simulink model "ebike"  (R2016a)
settings: Solver=ode3  StartTime=0.0  StopTime=1  FixedStep=0.001  MaxStep=0.001  MinStep=0.001  RelTol=1e-3
undefined symbols (not defined in the file or in its folder): RPM_motor_power
libraries: simulink x1
settings Model: Creator=stwei  LastModifiedBy=Aparajith Sridharan
settings DataIOCC: LimitDataPoints=on  SaveFormat=Array  SaveOutput=off  ReturnWorkspaceOutputs=on
settings OptimizationCC: ExpressionDepthLimit=2147483647
settings DebuggingCC: UnderspecifiedInitializationDetection=Classic  MergeDetectMultiDrivingBlocksExec=none  SolverPrmCheckMsg=warning  FcnCallInpInsideContextMsg=UseLocalSettings  StateNameClashWarn=warning
settings HardwareCC: ProdBitPerPointer=32  ProdLargestAtomicFloat=None  ProdIntDivRoundTo=Undefined  ProdEndianess=Unspecified  ProdWordSize=32  ProdHWDeviceType=32-bit Generic
settings ModelReferenceCC: PropagateSignalLabelsOutOfModel=off
settings GRTTargetCC: CombineOutputUpdateFcns=off  GRTInterface=on
settings ConfigComp: CovModelRefEnable=Off

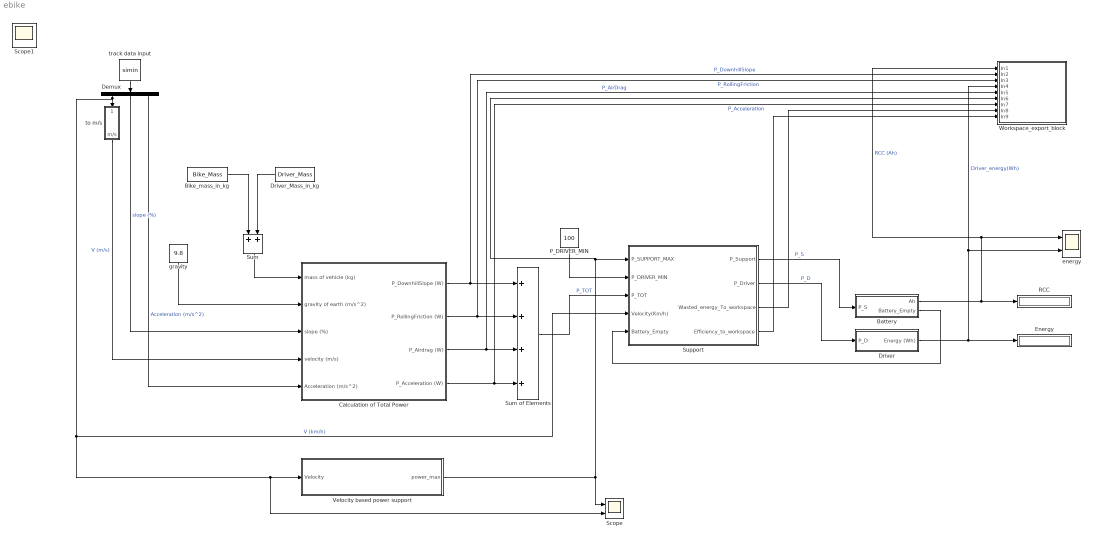
== system ebike ==
  Battery : Subsystem
  Bike_mass_in_kg : FromWorkspace  VariableName=Bike_Mass  SampleTime=0
  Calculation of Total Power : Subsystem
  Demux : Demux  Outputs=3
  Driver : Subsystem
  Driver_Mass_in_kg : FromWorkspace  VariableName=Driver_Mass  SampleTime=0
  Energy : Display
  P_DRIVER_MIN : Constant  Value=100
  RCC : Display
  Scope : Scope  NumInputPorts=2
  "Sum " : Sum
  Sum of Elements : Sum  Inputs=++++
  Support : Subsystem
  Velocity based power support : Subsystem
  Workspace_export_block : Subsystem
  energy : Scope  NumInputPorts=2
  gravity : Constant  Value=9.8
  to m/s : Subsystem
  track data input : FromWorkspace  VariableName=simin  SampleTime=0  OutputAfterFinalValue=Setting to zero
  Scope1 : Scope
  wires:
  P_DRIVER_MIN/1 -> Support/2(P_DRIVER_MIN)
  Support/2(P_Driver) -> Driver/1(P_D)  "P_D"
  Battery/1(Ah) -> RCC/1, energy/1, Workspace_export_block/1(In1)  "RCC (Ah)"
  track data input/1 -> Demux/1
  Demux/1 -> Support/4(Velocity(Km/h)), Scope/2, Velocity based power support/1(Velocity), to m/s/1(km/h)  "V (km/h)"
  Demux/2 -> Calculation of Total Power/3(slope (%))  "slope (%)"
  to m/s/1(m/s) -> Calculation of Total Power/4(velocity (m/s))  "V (m/s)"
  Sum of Elements/1 -> Support/3(P_TOT)  "P_TOT"
  Calculation of Total Power/1(P_DownhillSlope (W)) -> Workspace_export_block/2(In2), Sum of Elements/1  "P_DownhillSlope"
  Calculation of Total Power/2(P_RollingFriction (W)) -> Workspace_export_block/3(In3), Sum of Elements/2  "P_RollingFriction"
  Calculation of Total Power/3(P_Airdrag (W)) -> Workspace_export_block/5(In5), Sum of Elements/3  "P_AirDrag"
  Calculation of Total Power/4(P_Acceleration (W)) -> Workspace_export_block/7(In7), Sum of Elements/4  "P_Acceleration"
  gravity/1 -> Calculation of Total Power/2("gravity of earth (m/s^2) ")
  "Sum "/1 -> Calculation of Total Power/1(mass of vehicle (kg))
  Driver_Mass_in_kg/1 -> "Sum "/2
  Bike_mass_in_kg/1 -> "Sum "/1
  Demux/3 -> Calculation of Total Power/5(Acceleration (m/s^2))  "Acceleration (m/s^2)"
  Velocity based power support/1(power_max) -> Workspace_export_block/6(In6), Support/1(P_SUPPORT_MAX), Scope/1
  Driver/1(Energy (Wh)) -> Workspace_export_block/4(In4), energy/2, Energy/1  "Driver_energy(Wh)"
  Support/1(P_Support) -> Battery/1(P_S)  "P_S"
  Battery/2(Battery_Empty) -> Support/5(Battery_Empty)
  Support/3(Wasted_energy_To_workspace) -> Workspace_export_block/8(In8)
  Support/4(Efficiency_to_workspace) -> Workspace_export_block/9(In9)

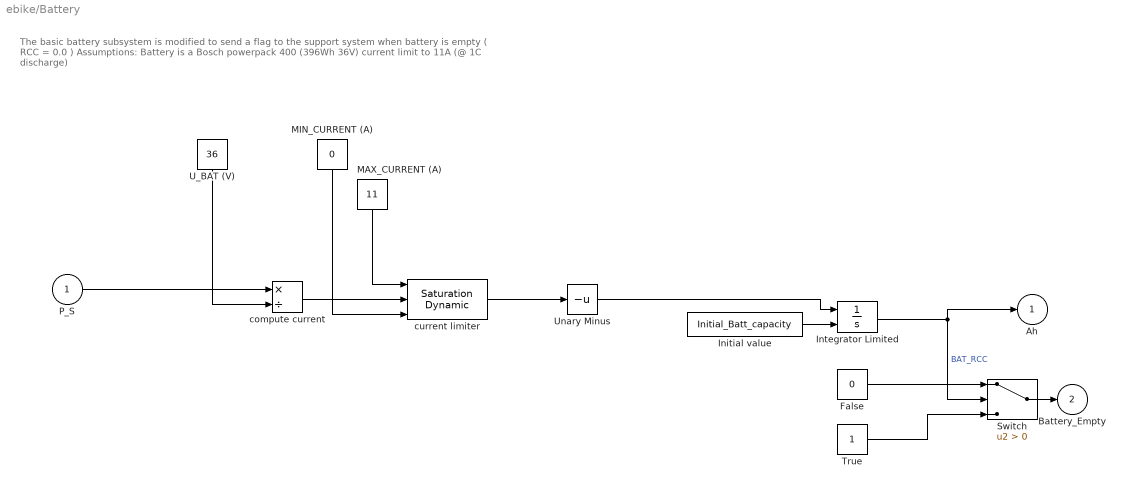
== system ebike/Battery ==
  note: The basic battery subsystem is modified to send a flag to the support system when battery is empty ( RCC = 0.0 )
      | Assumptions:
      | Battery is a Bosch powerpack 400 (396Wh 36V)
      | current limit to 11A (@ 1C discharge)
  P_S : Inport
  False : Constant  Value=0
  "Initial value " : FromWorkspace  VariableName=Initial_Batt_capacity  SampleTime=0
  Integrator Limited : Integrator  InitialConditionSource=external  LimitOutput=on  UpperSaturationLimit=11  LowerSaturationLimit=0
  MAX_CURRENT (A) : Constant  Value=11
  MIN_CURRENT (A) : Constant  Value=0
  Switch : Switch  Criteria=u2 > Threshold
  True : Constant
  U_BAT (V) : Constant  Value=36
  Unary Minus : UnaryMinus
  compute current : Product  Inputs=*/
  current limiter : simulink/Discontinuities/Saturation Dynamic  OutMin=[]  OutMax=[]  OutDataTypeStr=Inherit: Same as second input  OutDataType=fixdt(1, 16)  OutScaling=2^-10  DoSatur=on
  Ah : Outport
  Battery_Empty : Outport  Port=2
  wires:
  U_BAT (V)/1 -> compute current/2
  Integrator Limited/1 -> Ah/1, Switch/2  "BAT_RCC"
  current limiter/1 -> Unary Minus/1
  compute current/1 -> current limiter/2
  MAX_CURRENT (A)/1 -> current limiter/1
  MIN_CURRENT (A)/1 -> current limiter/3
  Unary Minus/1 -> Integrator Limited/1
  P_S/1 -> compute current/1
  "Initial value "/1 -> Integrator Limited/2
  Switch/1 -> Battery_Empty/1
  False/1 -> Switch/1
  True/1 -> Switch/3

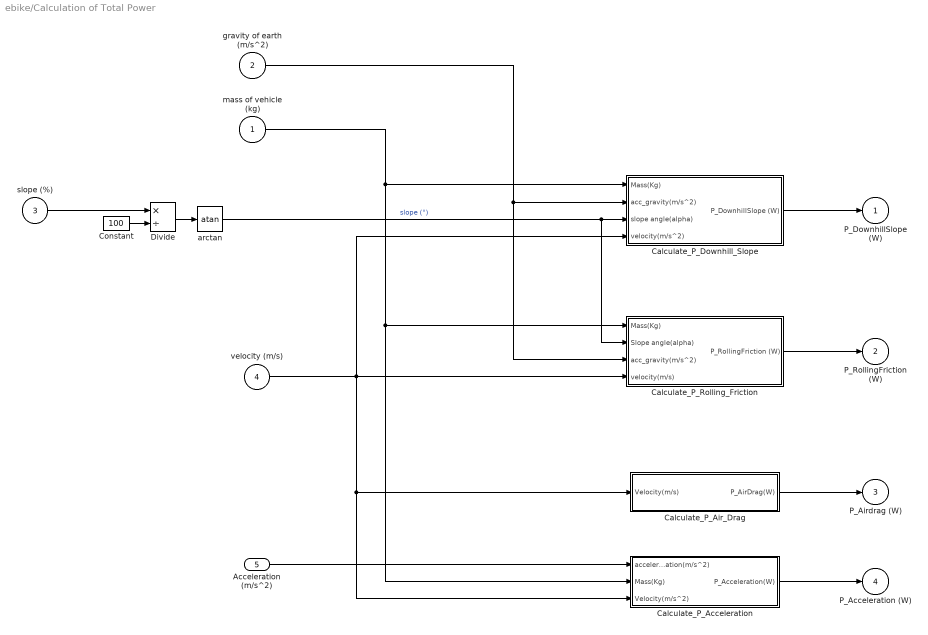
== system ebike/Calculation of Total Power ==
  mass of vehicle (kg) : Inport
  "gravity of earth (m/s^2) " : Inport  Port=2
  slope (%) : Inport  Port=3
  velocity (m/s) : Inport  Port=4
  Acceleration (m/s^2) : Inport  Port=5
  Calculate_P_Acceleration : Subsystem
  Calculate_P_Air_Drag : Subsystem
  Calculate_P_Downhill_Slope : Subsystem
  Calculate_P_Rolling_Friction : Subsystem
  Constant : Constant  Value=100
  Divide : Product  Inputs=*/
  arctan : Trigonometry  Operator=atan
  P_DownhillSlope (W) : Outport
  P_RollingFriction (W) : Outport  Port=2
  P_Airdrag (W) : Outport  Port=3
  P_Acceleration (W) : Outport  Port=4
  wires:
  mass of vehicle (kg)/1 -> Calculate_P_Downhill_Slope/1(Mass(Kg)), Calculate_P_Acceleration/2(Mass(Kg)), Calculate_P_Rolling_Friction/1(Mass(Kg))
  "gravity of earth (m/s^2) "/1 -> Calculate_P_Downhill_Slope/2(acc_gravity(m/s^2)), Calculate_P_Rolling_Friction/3(acc_gravity(m/s^2))
  velocity (m/s)/1 -> Calculate_P_Rolling_Friction/4(velocity(m/s)), Calculate_P_Air_Drag/1(Velocity(m/s)), Calculate_P_Acceleration/3(Velocity(m/s^2)), Calculate_P_Downhill_Slope/4(velocity(m/s^2))
  Calculate_P_Downhill_Slope/1(P_DownhillSlope (W)) -> P_DownhillSlope (W)/1
  arctan/1 -> Calculate_P_Rolling_Friction/2(Slope angle(alpha)), Calculate_P_Downhill_Slope/3(slope angle(alpha))  "slope (°)"
  Divide/1 -> arctan/1
  slope (%)/1 -> Divide/1
  Constant/1 -> Divide/2
  Acceleration (m/s^2)/1 -> Calculate_P_Acceleration/1(acceleration(m/s^2))
  Calculate_P_Acceleration/1("P_Acceleration(W) ") -> P_Acceleration (W)/1
  Calculate_P_Rolling_Friction/1(P_RollingFriction (W)) -> P_RollingFriction (W)/1
  Calculate_P_Air_Drag/1("P_AirDrag(W) ") -> P_Airdrag (W)/1

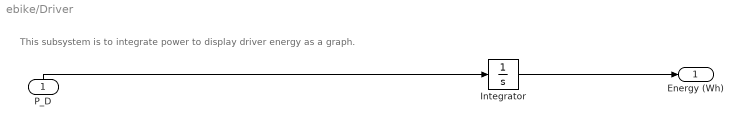
== system ebike/Driver ==
  note: This subsystem is to integrate power to display driver energy as a graph.
  P_D : Inport
  "Integrator " : Integrator  UpperSaturationLimit=400  LowerSaturationLimit=0
  Energy (Wh) : Outport
  wires:
  "Integrator "/1 -> Energy (Wh)/1
  P_D/1 -> "Integrator "/1

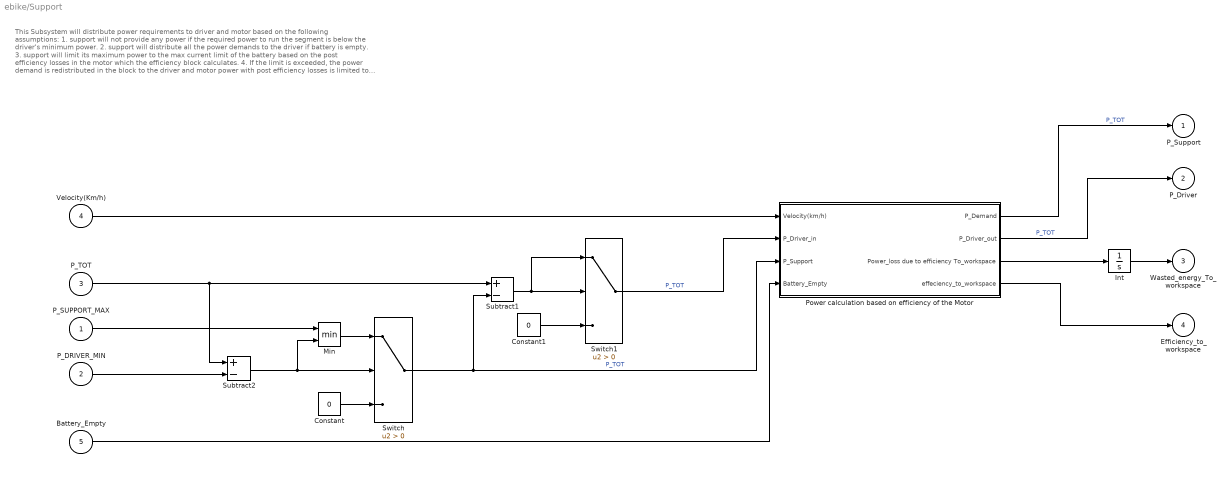
== system ebike/Support ==
  note: This Subsystem will distribute power requirements to driver and motor based on the following assumptions:
      | 1. support will not provide any power if the required power to run the segment is below the driver's minimum power.
      | 2. support will distribute all the power demands to the driver if battery is empty.
      | 3. support will limit its maximum power to the max current limit of the battery based on the post efficiency losses in the motor which the efficiency block calculates.
      | 4. If the limit is exceeded, the power demand is redistributed in the block to the driver and motor power with post efficiency losses is limited to max current limit of battery subsystem.
  P_SUPPORT_MAX : Inport
  P_DRIVER_MIN : Inport  Port=2
  P_TOT : Inport  Port=3
  Velocity(Km/h) : Inport  Port=4
  Battery_Empty : Inport  Port=5
  Constant : Constant  Value=0
  Constant1 : Constant  Value=0
  Int : Integrator
  Min : MinMax  Inputs=2
  Power calculation based on efficiency of the Motor : Subsystem
  Subtract1 : Sum  Inputs=+-
  Subtract2 : Sum  Inputs=+-
  Switch : Switch  Criteria=u2 > Threshold
  Switch1 : Switch  Criteria=u2 > Threshold
  P_Support : Outport
  P_Driver : Outport  Port=2
  Wasted_energy_To_workspace : Outport  Port=3
  Efficiency_to_workspace : Outport  Port=4
  wires:
  P_TOT/1 -> Subtract1/1, Subtract2/1
  Subtract2/1 -> Min/2, Switch/2
  P_SUPPORT_MAX/1 -> Min/1
  P_DRIVER_MIN/1 -> Subtract2/2
  Min/1 -> Switch/1
  Constant/1 -> Switch/3
  Constant1/1 -> Switch1/3
  Subtract1/1 -> Switch1/1, Switch1/2
  Velocity(Km/h)/1 -> Power calculation based on efficiency of the Motor/1(Velocity(km/h))
  Battery_Empty/1 -> Power calculation based on efficiency of the Motor/4(Battery_Empty)
  Switch/1 -> Power calculation based on efficiency of the Motor/3(P_Support), Subtract1/2  "P_TOT"
  Switch1/1 -> Power calculation based on efficiency of the Motor/2(P_Driver_in)  "P_TOT"
  Power calculation based on efficiency of the Motor/1(P_Demand) -> P_Support/1  "P_TOT"
  Power calculation based on efficiency of the Motor/2(P_Driver_out) -> P_Driver/1  "P_TOT"
  Int/1 -> Wasted_energy_To_workspace/1
  Power calculation based on efficiency of the Motor/3(Power_loss due to efficiency To_workspace) -> Int/1
  Power calculation based on efficiency of the Motor/4(effeciency_to_workspace) -> Efficiency_to_workspace/1

== system ebike/Velocity based power support ==
  note: This Subsystem will calculate the maximum power with respect to the current velocity of the system as a linear function.
      | power_max = { 0 : Velocity > 25
      | 250: Velocity < 22
      | (250/(3))*(25 - Velocity) : others}
  Velocity : Inport
  Calc_power_needed : MATLABFcn  MATLABFcn=calcpow  OutputDimensions=1
  power_max : Outport
  wires:
  Velocity/1 -> Calc_power_needed/1
  Calc_power_needed/1 -> power_max/1

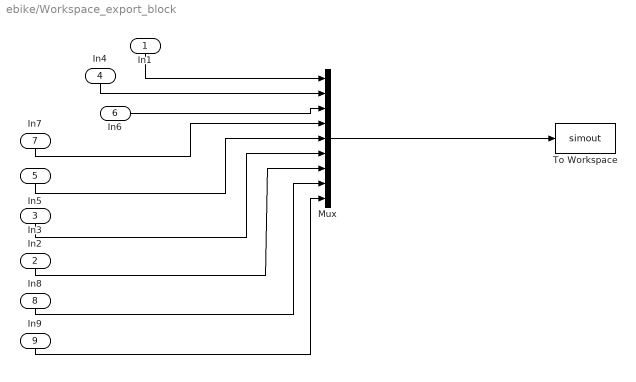
== system ebike/Workspace_export_block ==
  In1 : Inport
  In2 : Inport  Port=2
  In3 : Inport  Port=3
  In4 : Inport  Port=4
  In5 : Inport  Port=5
  In6 : Inport  Port=6
  In7 : Inport  Port=7
  In8 : Inport  Port=8
  In9 : Inport  Port=9
  Mux : Mux  Inputs=9
  To Workspace : ToWorkspace  VariableName=simout  SaveFormat=Timeseries  SampleTime=-1
  wires:
  Mux/1 -> To Workspace/1
  In6/1 -> Mux/3
  In5/1 -> Mux/5
  In3/1 -> Mux/6
  In4/1 -> Mux/2
  In2/1 -> Mux/7
  In1/1 -> Mux/1
  In7/1 -> Mux/4
  In8/1 -> Mux/8
  In9/1 -> Mux/9

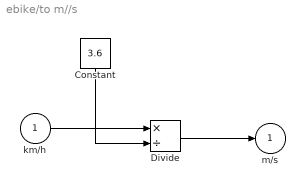
== system ebike/to m//s ==
  km/h : Inport
  Constant : Constant  Value=3.6
  Divide : Product  Inputs=*/
  m/s : Outport
  wires:
  Constant/1 -> Divide/2
  km/h/1 -> Divide/1
  Divide/1 -> m/s/1

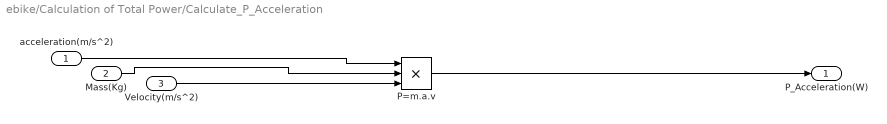
== system ebike/Calculation of Total Power/Calculate_P_Acceleration ==
  acceleration(m/s^2) : Inport
  Mass(Kg) : Inport  Port=2
  Velocity(m/s^2) : Inport  Port=3
  P=m.a.v : Product  Inputs=3
  "P_Acceleration(W) " : Outport
  wires:
  acceleration(m/s^2)/1 -> P=m.a.v/1
  P=m.a.v/1 -> "P_Acceleration(W) "/1
  Mass(Kg)/1 -> P=m.a.v/2
  Velocity(m/s^2)/1 -> P=m.a.v/3

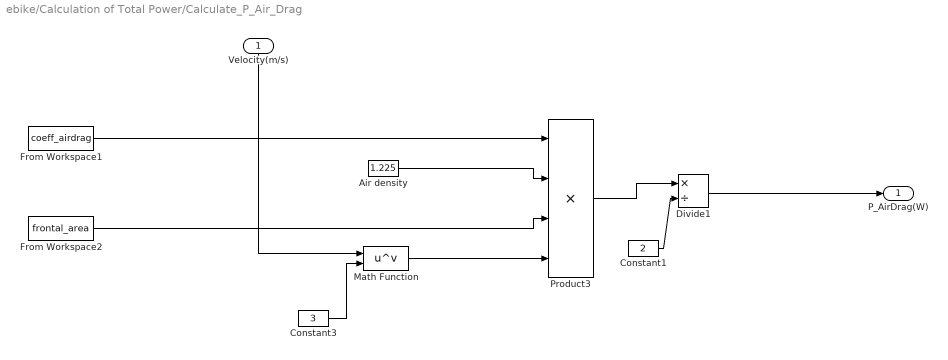
== system ebike/Calculation of Total Power/Calculate_P_Air_Drag ==
  Velocity(m/s) : Inport
  Air density : Constant  Value=1.225
  Constant1 : Constant  Value=2
  Constant3 : Constant  Value=3
  Divide1 : Product  Inputs=*/  SaturateOnIntegerOverflow=on  RndMeth=Zero
  From Workspace1 : FromWorkspace  VariableName=coeff_airdrag  SampleTime=0
  From Workspace2 : FromWorkspace  VariableName=frontal_area  SampleTime=0
  Math Function : Math  Operator=pow  SaturateOnIntegerOverflow=on
  Product3 : Product  Inputs=4
  "P_AirDrag(W) " : Outport
  wires:
  Air density/1 -> Product3/2
  Constant3/1 -> Math Function/2
  Divide1/1 -> "P_AirDrag(W) "/1
  Constant1/1 -> Divide1/2
  Math Function/1 -> Product3/4
  Product3/1 -> Divide1/1
  From Workspace1/1 -> Product3/1
  From Workspace2/1 -> Product3/3
  Velocity(m/s)/1 -> Math Function/1

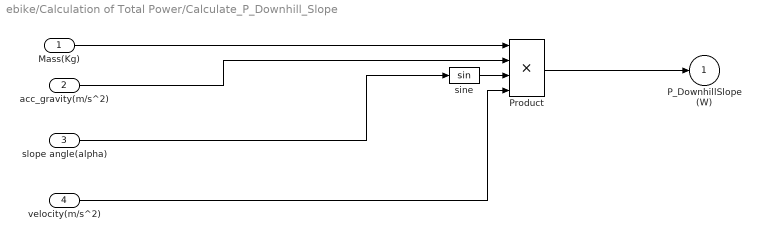
== system ebike/Calculation of Total Power/Calculate_P_Downhill_Slope ==
  Mass(Kg) : Inport
  acc_gravity(m/s^2) : Inport  Port=2
  slope angle(alpha) : Inport  Port=3
  velocity(m/s^2) : Inport  Port=4
  Product : Product  Inputs=4
  sine : Trigonometry
  P_DownhillSlope (W) : Outport
  wires:
  sine/1 -> Product/3
  Product/1 -> P_DownhillSlope (W)/1
  Mass(Kg)/1 -> Product/1
  velocity(m/s^2)/1 -> Product/4
  acc_gravity(m/s^2)/1 -> Product/2
  slope angle(alpha)/1 -> sine/1

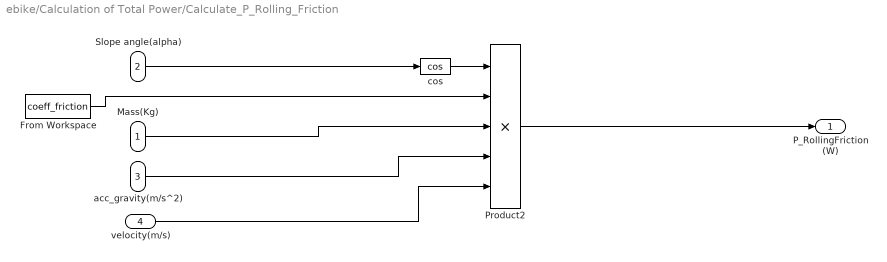
== system ebike/Calculation of Total Power/Calculate_P_Rolling_Friction ==
  Mass(Kg) : Inport
  Slope angle(alpha) : Inport  Port=2
  acc_gravity(m/s^2) : Inport  Port=3
  velocity(m/s) : Inport  Port=4
  From Workspace : FromWorkspace  VariableName=coeff_friction  SampleTime=0
  Product2 : Product  Inputs=5
  cos : Trigonometry  Operator=cos
  P_RollingFriction (W) : Outport
  wires:
  cos/1 -> Product2/1
  Product2/1 -> P_RollingFriction (W)/1
  From Workspace/1 -> Product2/2
  velocity(m/s)/1 -> Product2/5
  acc_gravity(m/s^2)/1 -> Product2/4
  Slope angle(alpha)/1 -> cos/1
  Mass(Kg)/1 -> Product2/3

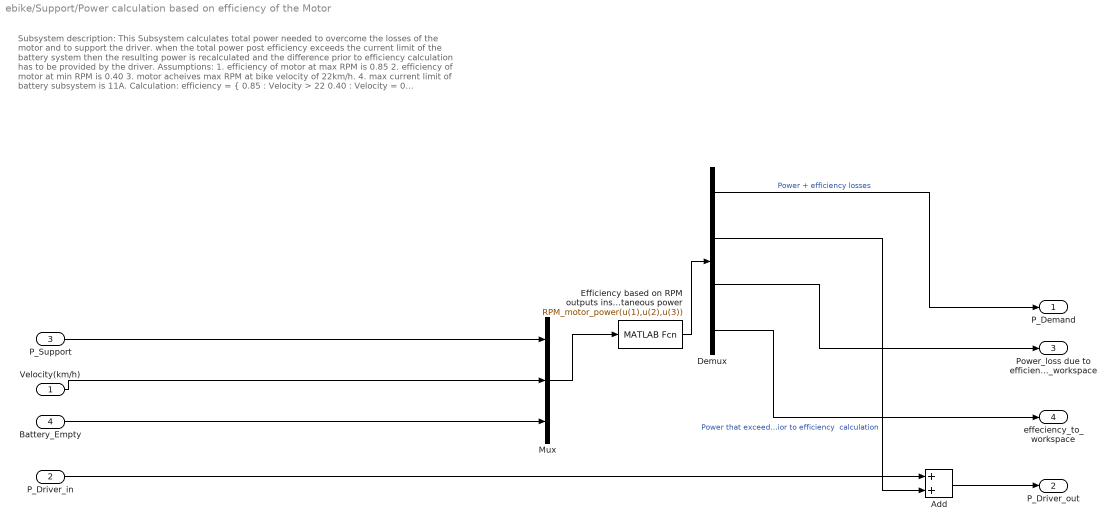
== system ebike/Support/Power calculation based on efficiency of the Motor ==
  note: Subsystem description:
      | This Subsystem calculates total power needed to overcome the losses of the motor and to support the driver.
      | when the total power post efficiency exceeds the current limit of the battery system then the resulting power
      | is recalculated and the difference prior to efficiency calculation has to be provided by the driver.
      |
      | Assumptions:
      | 1. efficiency of motor at max RPM is 0.85
      | 2. efficiency of motor at min RPM is 0.40
      | 3. motor acheives max RPM at bike velocity of 22km/h.
      | 4. max current limit of battery subsystem is 11A.
      |
      | Calculation:
      | efficiency = { 0.85 : Velocity > 22
      | 0.40 : Velocity = 0
      | (0.45/22)*Velocity + 0.40 : others }
  Velocity(km/h) : Inport
  P_Driver_in : Inport  Port=2
  P_Support : Inport  Port=3
  Battery_Empty : Inport  Port=4
  Add : Sum
  Demux : Demux
  Efficiency based on RPM outputs instantaneous power : MATLABFcn  MATLABFcn=RPM_motor_power(u(1),u(2),u(3))  Output1D=off
  Mux : Mux  Inputs=3
  P_Demand : Outport
  P_Driver_out : Outport  Port=2
  Power_loss due to efficiency To_workspace : Outport  Port=3
  effeciency_to_workspace : Outport  Port=4
  wires:
  P_Support/1 -> Mux/1
  Demux/1 -> P_Demand/1  "Power + efficiency losses"
  Efficiency based on RPM outputs instantaneous power/1 -> Demux/1
  Demux/2 -> Add/2  "Power that exceeds current limit.  prior to efficiency  calculation"
  Mux/1 -> Efficiency based on RPM outputs instantaneous power/1
  Velocity(km/h)/1 -> Mux/2
  Add/1 -> P_Driver_out/1
  P_Driver_in/1 -> Add/1
  Battery_Empty/1 -> Mux/3
  Demux/3 -> Power_loss due to efficiency To_workspace/1
  Demux/4 -> effeciency_to_workspace/1
